simulink subsystem "Control_Leds"  (R2023b)
settings: Solver=VariableStepAuto  StartTime=0.0  StopTime=10.0  RelTol=1e-3
libraries: simulink x2
settings Model: Creator=Felix  LastModifiedBy=Felix

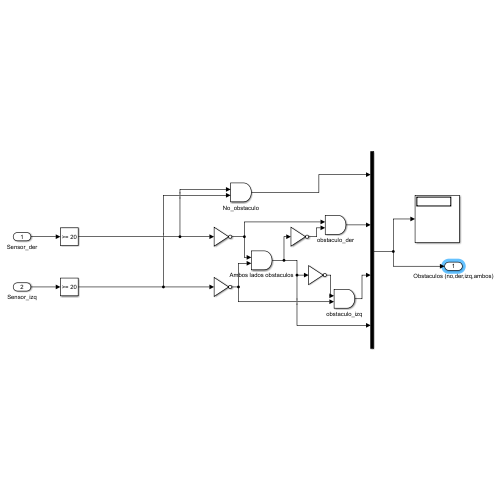
[thumbnail: Simulink's stored preview of the top-level diagram]
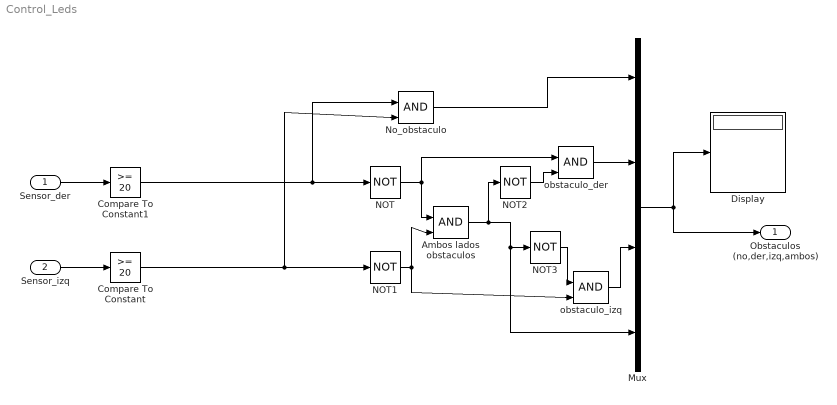
== system Control_Leds ==
  Sensor_der : Inport
  Sensor_izq : Inport  Port=2
  Ambos lados obstaculos : Logic  IconShape=distinctive  AllPortsSameDT=off  OutDataTypeStr=boolean
  Compare To Constant : simulink/Logic and Bit Operations/Compare To Constant  relop=>=  const=20  OutDataTypeStr=boolean
  Compare To Constant1 : simulink/Logic and Bit Operations/Compare To Constant  relop=>=  const=20  OutDataTypeStr=boolean
  Display : Display
  Mux : Mux
  NOT{,1..3} (4 alike) : Logic  Operator=NOT  IconShape=distinctive  AllPortsSameDT=off  OutDataTypeStr=boolean
  No_obstaculo : Logic  IconShape=distinctive  AllPortsSameDT=off  OutDataTypeStr=boolean
  obstaculo_der : Logic  IconShape=distinctive  AllPortsSameDT=off  OutDataTypeStr=boolean
  obstaculo_izq : Logic  IconShape=distinctive  AllPortsSameDT=off  OutDataTypeStr=boolean
  Obstaculos (no,der,izq,ambos) : Outport
  wires:
  NOT1/1 -> obstaculo_izq/2, Ambos lados obstaculos/2
  No_obstaculo/1 -> Mux/1
  obstaculo_der/1 -> Mux/2
  Ambos lados obstaculos/1 -> NOT2/1, Mux/4, NOT3/1
  NOT2/1 -> obstaculo_der/2
  obstaculo_izq/1 -> Mux/3
  Sensor_izq/1 -> Compare To Constant/1
  NOT/1 -> Ambos lados obstaculos/1, obstaculo_der/1
  NOT3/1 -> obstaculo_izq/1
  Compare To Constant/1 -> NOT1/1, No_obstaculo/2
  Mux/1 -> Obstaculos (no,der,izq,ambos)/1, Display/1
  Sensor_der/1 -> Compare To Constant1/1
  Compare To Constant1/1 -> NOT/1, No_obstaculo/1
